simulink model "EV_regenerative_braking_model"  (R2024b)
settings: Solver=ode45  StartTime=0.0  StopTime=25  RelTol=1e-3
model workspace (MAT data in the model file):
  Cd = Simulink.Parameter
  Cd.Value = 0.28
  Cd.Complexity = 'real'
  Cd.Dimensions = [1 1]
  Cd.DataType = 'auto'
  frontal_area = Simulink.Parameter
  frontal_area.Value = 2.2
  frontal_area.Complexity = 'real'
  frontal_area.Dimensions = [1 1]
  frontal_area.DataType = 'auto'
  rho_air = Simulink.Parameter
  rho_air.Value = 1.225
  rho_air.Complexity = 'real'
  rho_air.Dimensions = [1 1]
  rho_air.DataType = 'auto'
  vehicle_mass = Simulink.Parameter
  vehicle_mass.Value = 1200
  vehicle_mass.Complexity = 'real'
  vehicle_mass.Dimensions = [1 1]
  vehicle_mass.DataType = 'auto'
  vehicle_mass.DocUnits = 'kg'
  wheel_radius = Simulink.Parameter
  wheel_radius.Value = 0.3
  wheel_radius.Complexity = 'real'
  wheel_radius.Dimensions = [1 1]
  wheel_radius.DataType = 'auto'
libraries: simulink x2, SignalEditorBlockLib x1
settings Model: Creator=Shashwat Sinha  LastModifiedBy=Shashwat Sinha

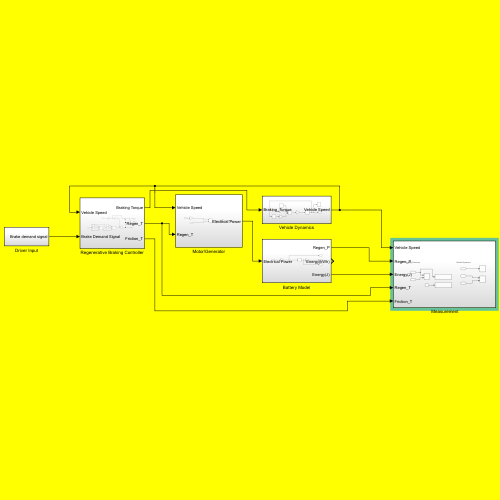
[thumbnail: Simulink's stored preview of the top-level diagram]
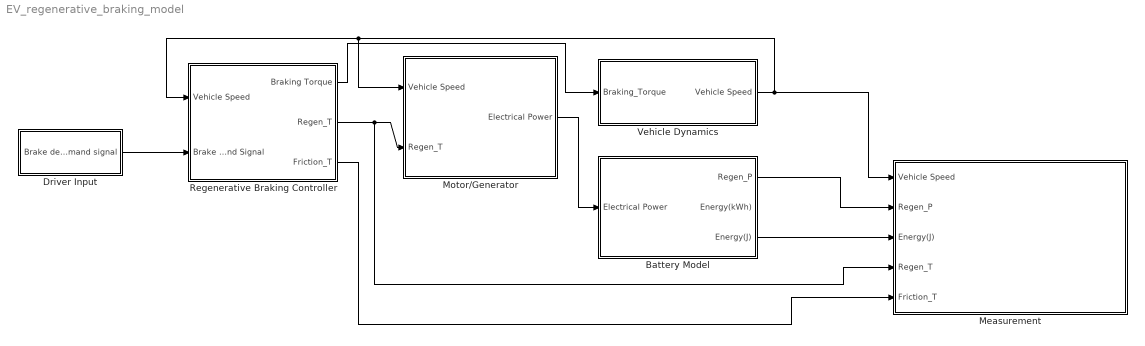
== system EV_regenerative_braking_model ==
  " Measurement" : Subsystem
  Battery Model : Subsystem
  Driver Input : Subsystem
  Motor/Generator : Subsystem
  Regenerative Braking Controller : Subsystem
  Vehicle Dynamics : Subsystem
  wires:
  Driver Input/1(Brake demand signal) -> Regenerative Braking Controller/2(Brake Demand Signal)
  Vehicle Dynamics/1(Vehicle Speed) -> Regenerative Braking Controller/1(Vehicle Speed), Motor/Generator/1(Vehicle Speed), " Measurement"/1(Vehicle Speed)
  Regenerative Braking Controller/2(Regen_T) -> " Measurement"/4(Regen_T), Motor/Generator/2(Regen_T)
  Motor/Generator/1(Electrical Power) -> Battery Model/1(Electrical Power)
  Regenerative Braking Controller/1(Braking Torque) -> Vehicle Dynamics/1(Braking_Torque)
  Battery Model/3(Energy(J)) -> " Measurement"/3(Energy(J))
  Battery Model/1(Regen_P) -> " Measurement"/2(Regen_P)
  Regenerative Braking Controller/3(Friction_T) -> " Measurement"/5(Friction_T)

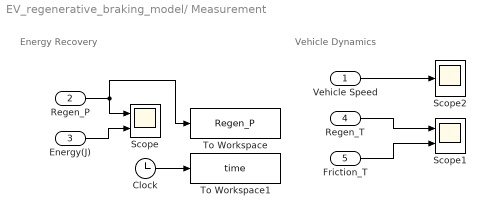
== system EV_regenerative_braking_model/ Measurement ==
  note: Energy Recovery
  note: Vehicle Dynamics
  Vehicle Speed : Inport
  Regen_P : Inport  Port=2
  Energy(J) : Inport  Port=3
  Regen_T : Inport  Port=4
  Friction_T : Inport  Port=5
  Clock : Clock
  Scope : Scope  NumInputPorts=2
  Scope1 : Scope  NumInputPorts=2
  Scope2 : Scope
  To Workspace : ToWorkspace  VariableName=Regen_P  SampleTime=-1
  To Workspace1 : ToWorkspace  VariableName=time  SampleTime=-1
  wires:
  Regen_P/1 -> Scope/1, To Workspace/1
  Energy(J)/1 -> Scope/2
  Regen_T/1 -> Scope1/1
  Friction_T/1 -> Scope1/2
  Vehicle Speed/1 -> Scope2/1
  Clock/1 -> To Workspace1/1

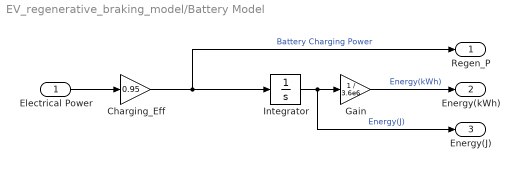
== system EV_regenerative_braking_model/Battery Model ==
  Electrical Power : Inport
  Charging_Eff : Gain  Gain=0.95
  Gain : Gain  Gain=1 / 3.6e6
  Integrator : Integrator
  Regen_P : Outport
  Energy(kWh) : Outport  Port=2
  Energy(J) : Outport  Port=3
  wires:
  Electrical Power/1 -> Charging_Eff/1
  Charging_Eff/1 -> Regen_P/1, Integrator/1  "Battery Charging Power"
  Integrator/1 -> Energy(J)/1, Gain/1  "Energy(J)"
  Gain/1 -> Energy(kWh)/1  "Energy(kWh)"

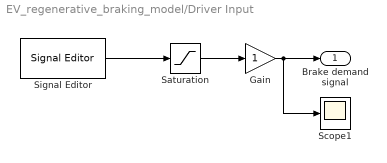
== system EV_regenerative_braking_model/Driver Input ==
  Gain : Gain
  Saturation : Saturate  UpperLimit=1  LowerLimit=0
  Scope1 : Scope
  Signal Editor : SignalEditorBlockLib/Signal Editor  FileName=D:\Regenerative Braking Model\Brake_Command_Signal.mat  ActiveScenario=Brake_Command  ActiveSignal=Signal 1  IsBus=off  OutputBusObjectStr=Bus: BusObject  SampleTime=0  ZeroCross=off  OutputAfterFinalValue=Setting to zero  Unit=inherit  PreserveSignalName=on  ApplySigPropsToAllScenarios=on  ApplySigPropsToAllSignals=off
  Brake demand signal : Outport
  wires:
  Signal Editor/1 -> Saturation/1
  Saturation/1 -> Gain/1
  Gain/1 -> Brake demand signal/1, Scope1/1

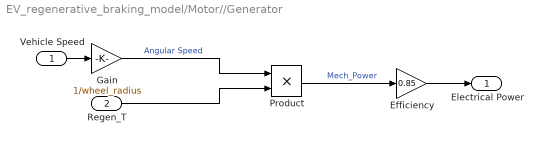
== system EV_regenerative_braking_model/Motor//Generator ==
  Vehicle Speed : Inport
  Regen_T : Inport  Port=2
  Efficiency : Gain  Gain=0.85
  Gain : Gain  Gain=1/wheel_radius
  Product : Product
  Electrical Power : Outport
  wires:
  Vehicle Speed/1 -> Gain/1
  Gain/1 -> Product/1  "Angular Speed"
  Regen_T/1 -> Product/2
  Product/1 -> Efficiency/1  "Mech_Power"
  Efficiency/1 -> Electrical Power/1

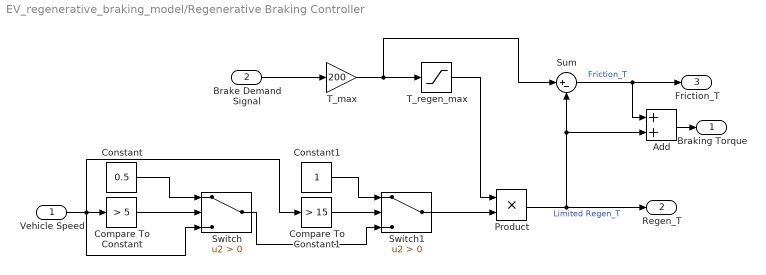
== system EV_regenerative_braking_model/Regenerative Braking Controller ==
  Vehicle Speed : Inport
  Brake Demand Signal : Inport  Port=2
  Add : Sum
  Compare To Constant : simulink/Logic and Bit Operations/Compare To Constant  relop=>  const=5  OutDataTypeStr=boolean
  Compare To Constant1 : simulink/Logic and Bit Operations/Compare To Constant  relop=>  const=15  OutDataTypeStr=boolean
  Constant : Constant  Value=0.5
  Constant1 : Constant
  Product : Product
  Sum : Sum  Inputs=|+-
  Switch : Switch  Criteria=u2 > Threshold  SaturateOnIntegerOverflow=off  InputSameDT=off
  Switch1 : Switch  Criteria=u2 > Threshold  SaturateOnIntegerOverflow=off  InputSameDT=off
  T_max : Gain  Gain=200
  T_regen_max : Saturate  UpperLimit=80  LowerLimit=0
  Braking Torque : Outport
  Regen_T : Outport  Port=2
  Friction_T : Outport  Port=3
  wires:
  Brake Demand Signal/1 -> T_max/1
  T_max/1 -> Sum/1, T_regen_max/1
  T_regen_max/1 -> Product/1
  Vehicle Speed/1 -> Switch/3, Compare To Constant1/1, Compare To Constant/1
  Constant/1 -> Switch/1
  Compare To Constant/1 -> Switch/2
  Switch/1 -> Switch1/3
  Constant1/1 -> Switch1/1
  Compare To Constant1/1 -> Switch1/2
  Switch1/1 -> Product/2
  Product/1 -> Add/2, Sum/2, Regen_T/1  "Limited Regen_T"
  Sum/1 -> Friction_T/1, Add/1  "Friction_T"
  Add/1 -> Braking Torque/1

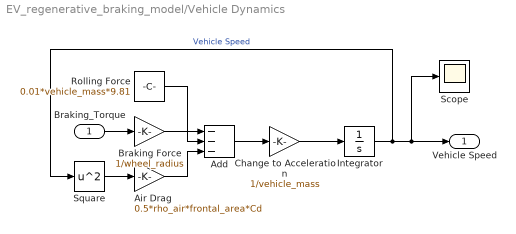
== system EV_regenerative_braking_model/Vehicle Dynamics ==
  Braking_Torque : Inport
  Add : Sum  Inputs=---
  Air Drag : Gain  Gain=0.5*rho_air*frontal_area*Cd
  Braking Force : Gain  Gain=1/wheel_radius
  Change to Acceleration : Gain  Gain=1/vehicle_mass
  Integrator : Integrator  InitialCondition=20
  Rolling Force : Constant  Value=0.01*vehicle_mass*9.81
  Scope : Scope
  Square : Math  Operator=square
  Vehicle Speed : Outport
  wires:
  Braking_Torque/1 -> Braking Force/1
  Braking Force/1 -> Add/1
  Rolling Force/1 -> Add/2
  Add/1 -> Change to Acceleration/1
  Change to Acceleration/1 -> Integrator/1
  Integrator/1 -> Square/1, Scope/1, Vehicle Speed/1  "Vehicle Speed"
  Square/1 -> Air Drag/1
  Air Drag/1 -> Add/3
